simulink model "controlador_multirate"  (R2012b)
settings: Solver=ode3  StartTime=0.0  StopTime=1  FixedStep=1e-5  RelTol=1e-6
undefined symbols (not defined in the file): J, Kd, Ke, Kt, L, P, R
libraries: simulink x45
(part 2 of 2)

== system controlador_multirate/Planta com o meu controlador discreto (calcula o Ts durante a execuçao)/Encoder/Método T ==
  A : Inport
  B : Inport  Port=2
  Posição : Inport  Port=3
  Add : Sum  Inputs=+-|
  Clock : Clock
  Compare To Constant : simulink/Logic and Bit Operations/Compare To Constant  relop===  const=m  OutDataTypeStr=boolean
  Contador : Subsystem
  Detect Change : simulink/Logic and Bit Operations/Detect Change  vinit=0  InputProcessing=Inherited  OutDataTypeStr=boolean
  Detect Change1 : simulink/Logic and Bit Operations/Detect Change  vinit=0  InputProcessing=Inherited  OutDataTypeStr=boolean
  Divide : Product  Inputs=*/
  Logical Operator : Logic  Operator=OR  AllPortsSameDT=off  OutDataTypeStr=boolean
  Memória controlavel : Subsystem
  Memória controlavel1 : Subsystem
  Sum : Sum  Inputs=|+-
  Switch1 : Switch
  pos' : Memory
  Velocidade : Outport
  wires:
  Posição/1 -> Add/1, Switch1/1
  Switch1/1 -> pos'/1
  pos'/1 -> Switch1/3, Add/2
  Memória controlavel1/1(Out) -> Velocidade/1
  Compare To Constant/1 -> Memória controlavel/2(ctrl), Switch1/2, Contador/2(reset), Memória controlavel1/2(ctrl)
  Clock/1 -> Memória controlavel/1(In), Sum/1
  Add/1 -> Divide/1
  Sum/1 -> Divide/2
  Memória controlavel/1(Out) -> Sum/2
  Divide/1 -> Memória controlavel1/1(In)
  Contador/1(Count) -> Compare To Constant/1
  Logical Operator/1 -> Contador/1(In)
  Detect Change1/1 -> Logical Operator/2
  Detect Change/1 -> Logical Operator/1
  B/1 -> Detect Change1/1
  A/1 -> Detect Change/1

== system controlador_multirate/Planta com o meu controlador discreto (calcula o Ts durante a execuçao)/Encoder/Sensor Óptico ==
  note: Saída do sensor óptico é:
      | 1, se	0 < mod(T,Tp) < \frac{Tp}{2}
      |  0, se      Tp/2 < mod(T,Tp) < Tp
  Theta : Inport
  Constant : Constant  Value=0
  Constant1 : Constant  Value=Nr
  Constant2 : Constant  Value=360
  Divide : Product  Inputs=*/
  Gain : Gain  Gain=1/2
  Logical Operator : Logic  AllPortsSameDT=off  OutDataTypeStr=boolean
  Math Function : Math  Operator=mod  SaturateOnIntegerOverflow=on
  Relational Operator : RelationalOperator  Operator=>  OutDataTypeStr=boolean
  Relational Operator1 : RelationalOperator  Operator=<  OutDataTypeStr=boolean
  Sinal_Pulso : Outport
  wires:
  Constant1/1 -> Divide/2
  Constant2/1 -> Divide/1
  Logical Operator/1 -> Sinal_Pulso/1
  Gain/1 -> Relational Operator1/2
  Divide/1 -> Gain/1, Math Function/2  "Theta_p"
  Constant/1 -> Relational Operator/2
  Relational Operator1/1 -> Logical Operator/2
  Relational Operator/1 -> Logical Operator/1
  Theta/1 -> Math Function/1
  Math Function/1 -> Relational Operator/1, Relational Operator1/1

== system controlador_multirate/Planta com o meu controlador discreto (calcula o Ts durante a execuçao)/Encoder/Sensor Óptico1 ==
  note: Saída do sensor óptico é:
      | 1, se	0 < mod(T-Tp/4,Tp) < Tp/2
      |  0, se     Tp/2 < mod(T-Tp/4,Tp) < Tp
  Theta : Inport
  Add : Sum  Inputs=+-
  Constant : Constant  Value=0
  Constant1 : Constant  Value=Nr
  Constant2 : Constant  Value=360
  Divide : Product  Inputs=*/
  Gain : Gain  Gain=1/2
  Gain1 : Gain  Gain=1/4
  Logical Operator : Logic  AllPortsSameDT=off  OutDataTypeStr=boolean
  Math Function : Math  Operator=mod  SaturateOnIntegerOverflow=on
  Relational Operator : RelationalOperator  Operator=>  OutDataTypeStr=boolean
  Relational Operator1 : RelationalOperator  Operator=<  OutDataTypeStr=boolean
  Sinal_Pulso : Outport
  wires:
  Gain1/1 -> Add/2
  Theta/1 -> Add/1
  Add/1 -> Math Function/1
  Math Function/1 -> Relational Operator1/1, Relational Operator/1
  Relational Operator/1 -> Logical Operator/1
  Relational Operator1/1 -> Logical Operator/2
  Constant/1 -> Relational Operator/2
  Divide/1 -> Math Function/2, Gain/1, Gain1/1  "Theta_p"
  Gain/1 -> Relational Operator1/2
  Logical Operator/1 -> Sinal_Pulso/1
  Constant2/1 -> Divide/1
  Constant1/1 -> Divide/2

== system controlador_multirate/Planta com o meu controlador discreto (calcula o Ts durante a execuçao)/Encoder/Subsystem ==
  note: Dependendo do sentido da rotaçao, incrementa ou decrementa o contador
  POS : Inport
  NEG : Inport  Port=2
  Constant : Constant  Value=4*Nr
  Conversion : DataTypeConversion  OutDataTypeStr=int32
  Conversion1 : DataTypeConversion  OutDataTypeStr=int32
  Math Function : Math  Operator=mod  SaturateOnIntegerOverflow=on
  Memory : Memory
  Sum : Sum  Inputs=+-+
  Out : Outport
  wires:
  NEG/1 -> Conversion1/1
  Conversion1/1 -> Sum/2
  Conversion/1 -> Sum/1
  POS/1 -> Conversion/1
  Math Function/1 -> Memory/1
  Memory/1 -> Sum/3, Out/1
  Sum/1 -> Math Function/1

== system controlador_multirate/Planta com o meu controlador discreto (calcula o Ts durante a execuçao)/Subsystem/Memória controlavel ==
  note: Memória controlável
      |
      | Se "ctrl" = 1, "Out" = "In"
      | Se "ctrl" = 0, "Out" mantém mesmo valor
  In : Inport
  ctrl : Inport  Port=2
  Memory2 : Memory
  Switch2 : Switch
  Out : Outport
  wires:
  Switch2/1 -> Memory2/1
  Memory2/1 -> Out/1, Switch2/3
  ctrl/1 -> Switch2/2
  In/1 -> Switch2/1

== system controlador_multirate/Planta com o meu controlador discreto (calcula o Ts durante a execuçao)/Subsystem/Memória controlavel (Y') ==
  note: Memória controlável
      |
      | Se "ctrl" = 1, "Out" = "In"
      | Se "ctrl" = 0, "Out" mantém mesmo valor
  In : Inport
  ctrl : Inport  Port=2
  Memory2 : Memory
  Switch2 : Switch
  Out : Outport
  wires:
  Switch2/1 -> Memory2/1
  Memory2/1 -> Out/1, Switch2/3
  ctrl/1 -> Switch2/2
  In/1 -> Switch2/1

== system controlador_multirate/Planta com o meu controlador discreto (calcula o Ts durante a execuçao)/Subsystem/Memória controlavel (e') ==
  note: Memória controlável
      |
      | Se "ctrl" = 1, "Out" = "In"
      | Se "ctrl" = 0, "Out" mantém mesmo valor
  In : Inport
  ctrl : Inport  Port=2
  Memory2 : Memory
  Switch2 : Switch
  Out : Outport
  wires:
  In/1 -> Switch2/1
  ctrl/1 -> Switch2/2
  Memory2/1 -> Switch2/3, Out/1
  Switch2/1 -> Memory2/1

== system controlador_multirate/Planta com o meu controlador discreto (calcula o Ts durante a execuçao)/Subsystem/Memória controlavel (u) ==
  note: Memória controlável
      |
      | Se "ctrl" = 1, "Out" = "In"
      | Se "ctrl" = 0, "Out" mantém mesmo valor
  In : Inport
  ctrl : Inport  Port=2
  Memory2 : Memory
  Switch2 : Switch
  Out : Outport
  wires:
  Switch2/1 -> Memory2/1
  Memory2/1 -> Out/1, Switch2/3
  ctrl/1 -> Switch2/2
  In/1 -> Switch2/1

== system controlador_multirate/Planta com controlador discreto do simulink/Encoder/Método T/Contador ==
  note: Contador de pulsos
      |
      | Conta o número de steps que a entrada "In" fica em nível lógico alto; reset em 1 zera.
      | Pode ser utilizado como contador se a entrada so ficar em nível alto por somente um
      | simulation step (por exemplo utilizando um bloco de "detect change").
  In : Inport
  reset : Inport  Port=2
  Constant : Constant  Value=0
  Constant1 : Constant
  Constant2 : Constant  Value=0
  Memory : Memory
  Sum : Sum  Inputs=|++
  Switch : Switch
  Switch1 : Switch
  Count : Outport
  wires:
  Constant/1 -> Switch/3
  Memory/1 -> Sum/1
  Constant1/1 -> Switch/1
  Sum/1 -> Switch1/3, Count/1
  Switch/1 -> Sum/2
  In/1 -> Switch/2
  reset/1 -> Switch1/2
  Constant2/1 -> Switch1/1
  Switch1/1 -> Memory/1

== system controlador_multirate/Planta com controlador discreto do simulink/Encoder/Método T/Memória controlavel ==
  note: Memória controlável
      |
      | Se "ctrl" = 1, "Out" = "In"
      | Se "ctrl" = 0, "Out" mantém mesmo valor
  In : Inport
  ctrl : Inport  Port=2
  Memory2 : Memory
  Switch2 : Switch
  Out : Outport
  wires:
  In/1 -> Switch2/1
  ctrl/1 -> Switch2/2
  Memory2/1 -> Switch2/3, Out/1
  Switch2/1 -> Memory2/1

== system controlador_multirate/Planta com controlador discreto do simulink/Encoder/Método T/Memória controlavel1 ==
  note: Memória controlável
      |
      | Se "ctrl" = 1, "Out" = "In"
      | Se "ctrl" = 0, "Out" mantém mesmo valor
  In : Inport
  ctrl : Inport  Port=2
  Memory2 : Memory
  Switch2 : Switch
  Out : Outport
  wires:
  Switch2/1 -> Memory2/1
  Memory2/1 -> Out/1, Switch2/3
  ctrl/1 -> Switch2/2
  In/1 -> Switch2/1

== system controlador_multirate/Planta com o meu controlador discreto (calcula o Ts durante a execuçao)/Encoder/Método T/Contador ==
  note: Contador de pulsos
      |
      | Conta o número de steps que a entrada "In" fica em nível lógico alto; reset em 1 zera.
      | Pode ser utilizado como contador se a entrada so ficar em nível alto por somente um
      | simulation step (por exemplo utilizando um bloco de "detect change").
  In : Inport
  reset : Inport  Port=2
  Constant : Constant  Value=0
  Constant1 : Constant
  Constant2 : Constant  Value=0
  Memory : Memory
  Sum : Sum  Inputs=|++
  Switch : Switch
  Switch1 : Switch
  Count : Outport
  wires:
  Constant/1 -> Switch/3
  Memory/1 -> Sum/1
  Constant1/1 -> Switch/1
  Sum/1 -> Switch1/3, Count/1
  Switch/1 -> Sum/2
  In/1 -> Switch/2
  reset/1 -> Switch1/2
  Constant2/1 -> Switch1/1
  Switch1/1 -> Memory/1

== system controlador_multirate/Planta com o meu controlador discreto (calcula o Ts durante a execuçao)/Encoder/Método T/Memória controlavel ==
  note: Memória controlável
      |
      | Se "ctrl" = 1, "Out" = "In"
      | Se "ctrl" = 0, "Out" mantém mesmo valor
  In : Inport
  ctrl : Inport  Port=2
  Memory2 : Memory
  Switch2 : Switch
  Out : Outport
  wires:
  In/1 -> Switch2/1
  ctrl/1 -> Switch2/2
  Memory2/1 -> Switch2/3, Out/1
  Switch2/1 -> Memory2/1

== system controlador_multirate/Planta com o meu controlador discreto (calcula o Ts durante a execuçao)/Encoder/Método T/Memória controlavel1 ==
  note: Memória controlável
      |
      | Se "ctrl" = 1, "Out" = "In"
      | Se "ctrl" = 0, "Out" mantém mesmo valor
  In : Inport
  ctrl : Inport  Port=2
  Memory2 : Memory
  Switch2 : Switch
  Out : Outport
  wires:
  Switch2/1 -> Memory2/1
  Memory2/1 -> Out/1, Switch2/3
  ctrl/1 -> Switch2/2
  In/1 -> Switch2/1
